simulink model "twsbr_attitude_pid"  (R2026a)
settings: Solver=ode45  StopTime=5.0  MaxStep=0.001  RelTol=1e-9  AbsTol=1e-11
model workspace (MAT data in the model file):
  force_disturbance_data = [0  0; 5  0]
  theta_reference_data = [0  0; 5  0]
  torque_disturbance_data = [0  0; 5  0]
settings Model: Creator=Linxiuqi  LastModifiedBy=Linxiuqi

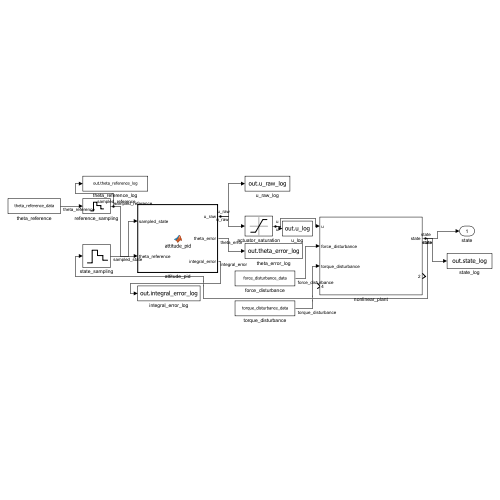
[thumbnail: Simulink's stored preview of the top-level diagram]
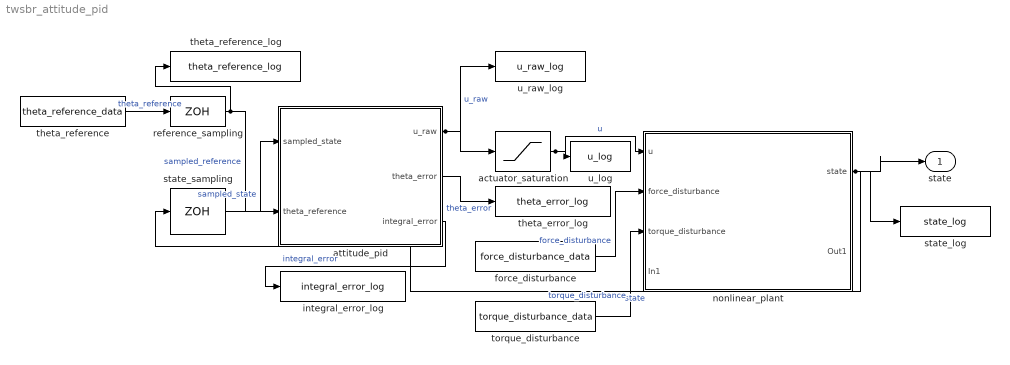
== system twsbr_attitude_pid ==
  actuator_saturation : Saturate  UpperLimit=1  LowerLimit=-1
  attitude_pid : MATLAB Function  TreatAsAtomicUnit=on
  force_disturbance : FromWorkspace  VariableName=force_disturbance_data  Interpolate=off  OutputAfterFinalValue=Holding final value
  integral_error_log : ToWorkspace  VariableName=integral_error_log  SaveFormat=Structure With Time  SampleTime=-1
  nonlinear_plant : Subsystem
  reference_sampling : ZeroOrderHold  SampleTime=0.01
  state_log : ToWorkspace  VariableName=state_log  SaveFormat=Structure With Time  SampleTime=-1
  state_sampling : ZeroOrderHold  SampleTime=0.01
  theta_error_log : ToWorkspace  VariableName=theta_error_log  SaveFormat=Structure With Time  SampleTime=-1
  theta_reference : FromWorkspace  VariableName=theta_reference_data  Interpolate=off  OutputAfterFinalValue=Holding final value
  theta_reference_log : ToWorkspace  VariableName=theta_reference_log  SaveFormat=Structure With Time  SampleTime=-1
  torque_disturbance : FromWorkspace  VariableName=torque_disturbance_data  Interpolate=off  OutputAfterFinalValue=Holding final value
  u_log : ToWorkspace  VariableName=u_log  SaveFormat=Structure With Time  SampleTime=-1
  u_raw_log : ToWorkspace  VariableName=u_raw_log  SaveFormat=Structure With Time  SampleTime=-1
  state : Outport
  wires:
  theta_reference/1 -> reference_sampling/1  "theta_reference"
  reference_sampling/1 -> attitude_pid/2(theta_reference), theta_reference_log/1  "sampled_reference"
  nonlinear_plant/1(state) -> state_sampling/1, state/1, state_log/1  "state"
  state_sampling/1 -> attitude_pid/1(sampled_state)  "sampled_state"
  attitude_pid/1(u_raw) -> actuator_saturation/1, u_raw_log/1  "u_raw"
  attitude_pid/2(theta_error) -> theta_error_log/1  "theta_error"
  attitude_pid/3(integral_error) -> integral_error_log/1  "integral_error"
  actuator_saturation/1 -> nonlinear_plant/1(u), u_log/1  "u"
  force_disturbance/1 -> nonlinear_plant/2(force_disturbance)  "force_disturbance"
  torque_disturbance/1 -> nonlinear_plant/3(torque_disturbance)  "torque_disturbance"

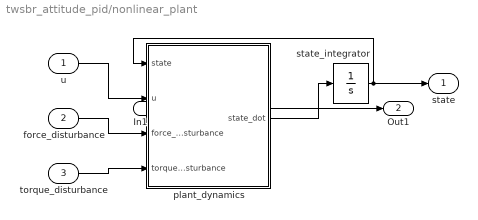
== system twsbr_attitude_pid/nonlinear_plant ==
  u : Inport
  force_disturbance : Inport  Port=2
  torque_disturbance : Inport  Port=3
  In1 : Inport  Port=4
  plant_dynamics : MATLAB Function  TreatAsAtomicUnit=on
  state_integrator : Integrator  InitialCondition=[0;0;0;0]
  state : Outport
  Out1 : Outport  Port=2
  wires:
  plant_dynamics/1(state_dot) -> state_integrator/1
  torque_disturbance/1 -> plant_dynamics/4(torque_disturbance)
  force_disturbance/1 -> plant_dynamics/3(force_disturbance)
  u/1 -> plant_dynamics/2(u)
  state_integrator/1 -> state/1, plant_dynamics/1(state)
  In1/1 -> Out1/1

== matlab function twsbr_attitude_pid/nonlinear_plant/plant_dynamics ==
  data: state input; u input; state_dot output; force_disturbance input; torque_disturbance input
function state_dot = plant_dynamics(state, u, force_disturbance, torque_disturbance)
%#codegen
body_mass = 1.2;
wheel_mass = 0.29999999999999999;
com_length = 0.17999999999999999;
body_inertia = 0.025000000000000001;
damping = 0.050000000000000003;
gravity = 9.8100000000000005;
motor_gain = 12;
x_dot = state(2);
theta = state(3);
theta_dot = state(4);
force = motor_gain * u + force_disturbance;
mass_sum = wheel_mass + body_mass;
rotational_term = body_inertia + body_mass * com_length^2;
coupling = body_mass * com_length * cos(theta);
rhs_position = force - damping * x_dot + body_mass * com_length * theta_dot^2 * sin(theta);
rhs_angle = body_mass * gravity * com_length * sin(theta) + torque_disturbance;
determinant = mass_sum * rotational_term - coupling^2;
x_ddot = (rotational_term * rhs_position - coupling * rhs_angle) / determinant;
theta_ddot = (-coupling * rhs_position + mass_sum * rhs_angle) / determinant;
state_dot = [x_dot; x_ddot; theta_dot; theta_ddot];
end

== matlab function twsbr_attitude_pid/attitude_pid ==
  data: sampled_state input; u_raw output; theta_reference input; theta_error output; integral_error output
function [u_raw, theta_error, integral_error] = attitude_pid(sampled_state, theta_reference)
%#codegen
persistent integral_state
if isempty(integral_state)
    integral_state = 0.0;
end
kp = 1.8999999999999999;
ki = 0.20000000000000001;
kd = 0.17999999999999999;
sample_time = 0.01;
integral_limit = 0.5;
u_max = 1;
theta = sampled_state(3);
theta_dot = sampled_state(4);
theta_error = theta - theta_reference;
u_raw = kp * theta_error + ki * integral_state + kd * theta_dot;
saturated = abs(u_raw) > u_max + 1.0e-12;
if ~saturated || theta_error * u_raw < 0.0
    integral_state = integral_state + sample_time * theta_error;
end
integral_state = min(max(integral_state, -integral_limit), integral_limit);
integral_error = integral_state;
end
